simulink model "Dynamic_Phasor_Extraction_SFA"  (R2021b)
settings: Solver=VariableStepAuto  StartTime=0.0  StopTime=10.0  RelTol=1e-3
undefined symbols (not defined in the file): j
libraries: eeGeneralControl x2
settings Model: Creator=Antero  LastModifiedBy=Antero

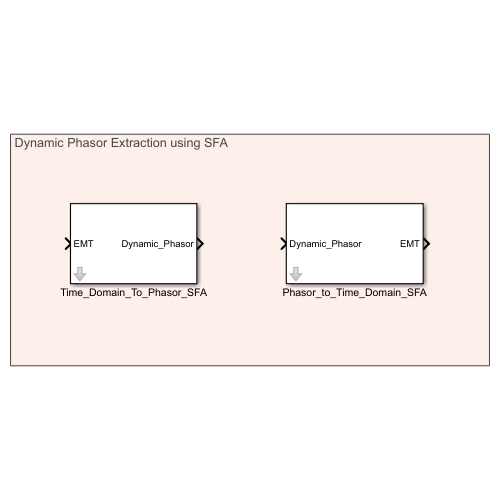
[thumbnail: Simulink's stored preview of the top-level diagram]
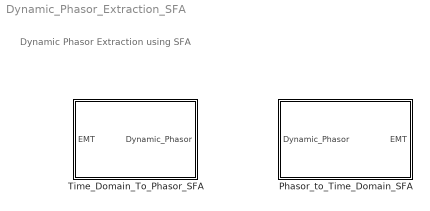
== system Dynamic_Phasor_Extraction_SFA ==
  note: Dynamic Phasor Extraction using SFA
  Phasor_to_Time_Domain_SFA : Subsystem  mask(Time domain from Dynamic Phasor){offset=60}
      mask prompts: offset "Frequency shift"
      mask help: This block extracts Time Domain Signals from the Dynamic Phasor by using the SFA method. It is usable only for three-phase signals
  Time_Domain_To_Phasor_SFA : Subsystem  mask(SFA){offset=60}
      mask prompts: offset "Frequency shift"
      mask help: This block extracts Dynamic Phasor by using the SFA method. It is usable only for three-phase signals

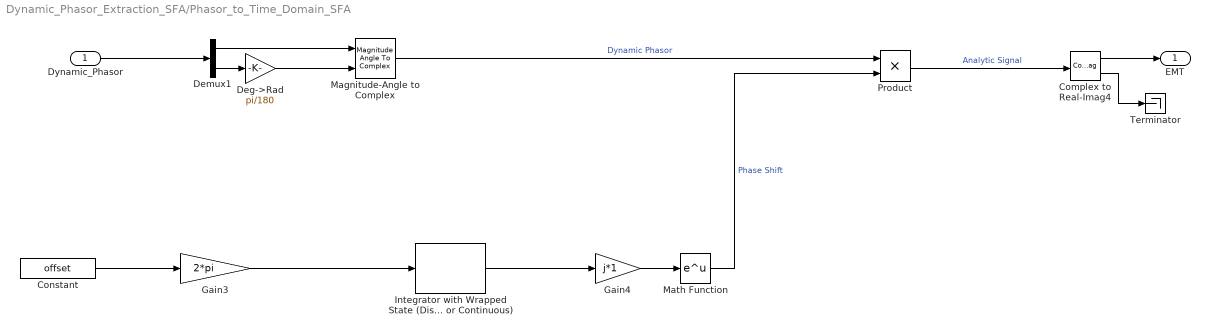
== system Dynamic_Phasor_Extraction_SFA/Phasor_to_Time_Domain_SFA ==
  Dynamic_Phasor : Inport
  Complex to Real-Imag4 : ComplexToRealImag
  Constant : Constant  Value=offset
  Deg->Rad : Gain  Gain=pi/180
  Demux1 : Demux  Outputs=2
  Gain3 : Gain  Gain=2*pi
  Gain4 : Gain  Gain=j*1
  Integrator with Wrapped State (Discrete or Continuous) : eeGeneralControl/Integrator with Wrapped State (Discrete or Continuous)  LabelModeActiveChoice=Discrete  WrappedStateUpperValue=2*pi  WrappedStateLowerValue=0  x0=0  Ts=-1
      settings: SourceProductBaseCode=PS
  Magnitude-Angle to Complex : MagnitudeAngleToComplex
  Math Function : Math  SaturateOnIntegerOverflow=on
  Product : Product
  Terminator : Terminator
  EMT : Outport
  wires:
  Dynamic_Phasor/1 -> Demux1/1
  Product/1 -> Complex to Real-Imag4/1  "Analytic Signal"
  Magnitude-Angle to Complex/1 -> Product/1  "Dynamic Phasor"
  Complex to Real-Imag4/2 -> Terminator/1
  Complex to Real-Imag4/1 -> EMT/1
  Demux1/1 -> Magnitude-Angle to Complex/1
  Demux1/2 -> Deg->Rad/1
  Deg->Rad/1 -> Magnitude-Angle to Complex/2
  Constant/1 -> Gain3/1
  Math Function/1 -> Product/2  "Phase Shift"
  Gain4/1 -> Math Function/1
  Gain3/1 -> Integrator with Wrapped State (Discrete or Continuous)/1
  Integrator with Wrapped State (Discrete or Continuous)/1 -> Gain4/1

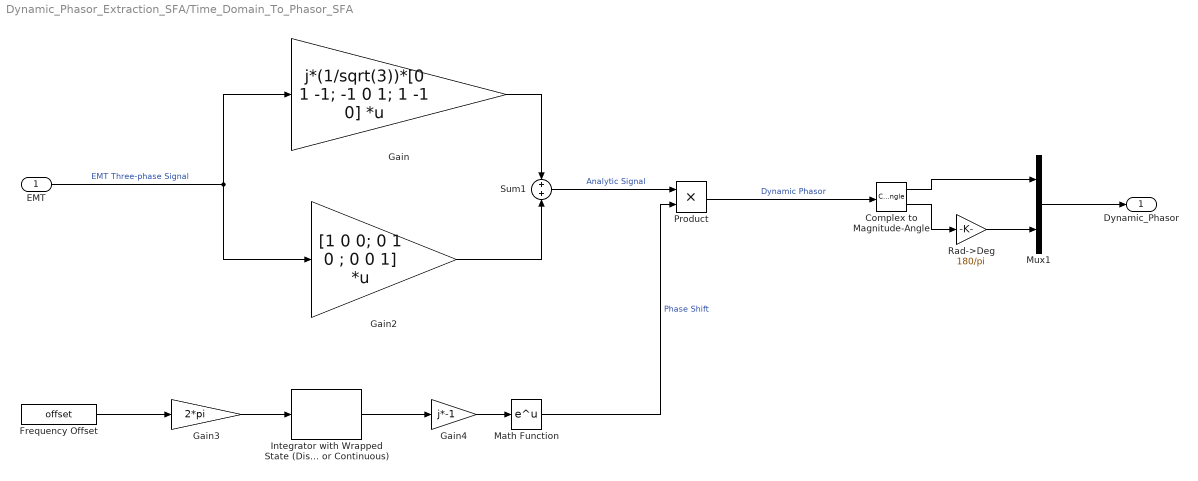
== system Dynamic_Phasor_Extraction_SFA/Time_Domain_To_Phasor_SFA ==
  EMT : Inport
  Complex to Magnitude-Angle : ComplexToMagnitudeAngle
  Frequency Offset : Constant  Value=offset
  Gain : Gain  Gain=j*(1/sqrt(3))*[0 1 -1; -1 0 1; 1 -1 0]  Multiplication=Matrix(K*u)
  Gain2 : Gain  Gain="[1  0 0; 0 1 0 ; 0 0 1]"  Multiplication=Matrix(K*u)
  Gain3 : Gain  Gain=2*pi
  Gain4 : Gain  Gain=j*-1
  Integrator with Wrapped State (Discrete or Continuous) : eeGeneralControl/Integrator with Wrapped State (Discrete or Continuous)  LabelModeActiveChoice=Discrete  WrappedStateUpperValue=2*pi  WrappedStateLowerValue=0  x0=0  Ts=-1
      settings: SourceProductBaseCode=PS
  Math Function : Math  SaturateOnIntegerOverflow=on
  Mux1 : Mux  Inputs=2
  Product : Product
  Rad->Deg : Gain  Gain=180/pi
  Sum1 : Sum  Inputs=+|+
  Dynamic_Phasor : Outport
  wires:
  Sum1/1 -> Product/1  "Analytic Signal"
  Mux1/1 -> Dynamic_Phasor/1
  Gain2/1 -> Sum1/2
  Complex to Magnitude-Angle/1 -> Mux1/1
  Gain/1 -> Sum1/1
  Rad->Deg/1 -> Mux1/2
  EMT/1 -> Gain/1, Gain2/1  "EMT Three-phase Signal"
  Product/1 -> Complex to Magnitude-Angle/1  "Dynamic Phasor"
  Complex to Magnitude-Angle/2 -> Rad->Deg/1
  Gain4/1 -> Math Function/1
  Frequency Offset/1 -> Gain3/1
  Math Function/1 -> Product/2  "Phase Shift"
  Gain3/1 -> Integrator with Wrapped State (Discrete or Continuous)/1
  Integrator with Wrapped State (Discrete or Continuous)/1 -> Gain4/1
